simulink model "TorqueVect_FS_with_kalmanFilter"  (R2022a)
settings: Solver=FixedStepAuto  StartTime=0.0  StopTime=inf  FixedStep=0.001  RelTol=1e-3  EnableMultiTasking=on
PreLoadFcn:
  | run('Parameters\FSE_Parameters.m')
libraries: CarMaker4SL x42, simulink x1
(part 3 of 3)

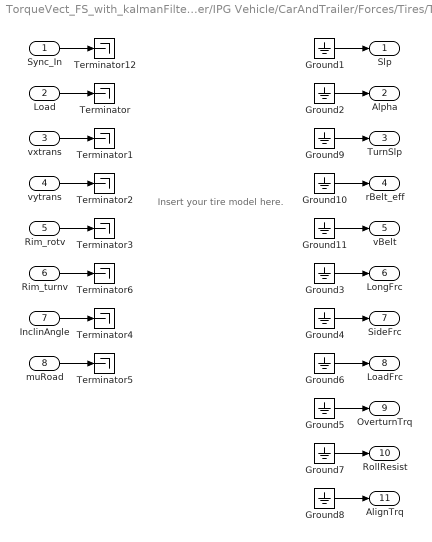
== system TorqueVect_FS_with_kalmanFilter/CarMaker/IPG Vehicle/CarAndTrailer/Forces/Tires/TireRL ==
  note: Insert your tire model here.
  Sync_In : Inport
  Load : Inport  Port=2
  vxtrans : Inport  Port=3
  vytrans : Inport  Port=4
  Rim_rotv : Inport  Port=5
  Rim_turnv : Inport  Port=6
  InclinAngle : Inport  Port=7
  muRoad : Inport  Port=8
  Ground{1..11} (11 alike) : Ground
  Terminator{,1..6,12} (8 alike) : Terminator
  Slp : Outport
  Alpha : Outport  Port=2
  TurnSlp : Outport  Port=3
  rBelt_eff : Outport  Port=4
  vBelt : Outport  Port=5
  LongFrc : Outport  Port=6
  SideFrc : Outport  Port=7
  LoadFrc : Outport  Port=8
  OverturnTrq : Outport  Port=9
  RollResist : Outport  Port=10
  AlignTrq : Outport  Port=11
  wires:
  Ground11/1 -> vBelt/1
  Ground10/1 -> rBelt_eff/1
  Ground9/1 -> TurnSlp/1
  Rim_turnv/1 -> Terminator6/1
  Sync_In/1 -> Terminator12/1
  Ground2/1 -> Alpha/1
  Ground3/1 -> LongFrc/1
  Ground4/1 -> SideFrc/1
  Ground5/1 -> OverturnTrq/1
  vxtrans/1 -> Terminator1/1
  vytrans/1 -> Terminator2/1
  Rim_rotv/1 -> Terminator3/1
  InclinAngle/1 -> Terminator4/1
  muRoad/1 -> Terminator5/1
  Load/1 -> Terminator/1
  Ground1/1 -> Slp/1
  Ground6/1 -> LoadFrc/1
  Ground7/1 -> RollResist/1
  Ground8/1 -> AlignTrq/1

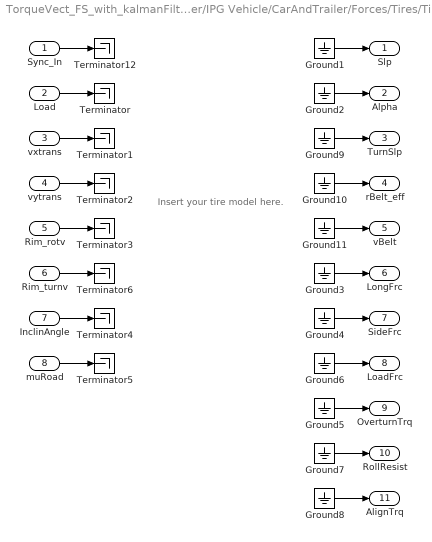
== system TorqueVect_FS_with_kalmanFilter/CarMaker/IPG Vehicle/CarAndTrailer/Forces/Tires/TireRR ==
  note: Insert your tire model here.
  Sync_In : Inport
  Load : Inport  Port=2
  vxtrans : Inport  Port=3
  vytrans : Inport  Port=4
  Rim_rotv : Inport  Port=5
  Rim_turnv : Inport  Port=6
  InclinAngle : Inport  Port=7
  muRoad : Inport  Port=8
  Ground{1..11} (11 alike) : Ground
  Terminator{,1..6,12} (8 alike) : Terminator
  Slp : Outport
  Alpha : Outport  Port=2
  TurnSlp : Outport  Port=3
  rBelt_eff : Outport  Port=4
  vBelt : Outport  Port=5
  LongFrc : Outport  Port=6
  SideFrc : Outport  Port=7
  LoadFrc : Outport  Port=8
  OverturnTrq : Outport  Port=9
  RollResist : Outport  Port=10
  AlignTrq : Outport  Port=11
  wires:
  Ground11/1 -> vBelt/1
  Ground10/1 -> rBelt_eff/1
  Ground9/1 -> TurnSlp/1
  Rim_turnv/1 -> Terminator6/1
  Sync_In/1 -> Terminator12/1
  Ground2/1 -> Alpha/1
  Ground3/1 -> LongFrc/1
  Ground4/1 -> SideFrc/1
  Ground5/1 -> OverturnTrq/1
  vxtrans/1 -> Terminator1/1
  vytrans/1 -> Terminator2/1
  Rim_rotv/1 -> Terminator3/1
  InclinAngle/1 -> Terminator4/1
  muRoad/1 -> Terminator5/1
  Load/1 -> Terminator/1
  Ground1/1 -> Slp/1
  Ground6/1 -> LoadFrc/1
  Ground7/1 -> RollResist/1
  Ground8/1 -> AlignTrq/1

== system TorqueVect_FS_with_kalmanFilter/CarMaker/IPG Vehicle/PowerTrain/PTControl Example/PTControl/Control_value ==
  ht : Inport
  lf : Inport  Port=2
  FL_Fx : Inport  Port=3
  FR_Fx : Inport  Port=4
  cos : Inport  Port=5
  sin : Inport  Port=6
  FR : Inport  Port=7
  In8 : Inport  Port=8
  Add{4..7} (4 alike) : Sum
  Minus : Sum  Inputs=+-
  Product{10..13,15..17} (7 alike) : Product
  Mx : Outport
  wires:
  Product10/1 -> Minus/1
  cos/1 -> Product10/2, Product11/1
  FR_Fx/1 -> Product13/2, Product11/2
  Product16/1 -> Add5/2
  sin/1 -> Product12/1, Product13/1
  Product17/1 -> Add5/1
  ht/1 -> Product15/1, Product17/1
  FL_Fx/1 -> Product10/1, Product12/2
  Add5/1 -> Add7/1
  Product12/1 -> Add4/1
  In8/1 -> Add6/2
  Product11/1 -> Minus/2
  Product13/1 -> Add4/2
  Product15/1 -> Add7/2
  Add4/1 -> Product16/2
  Add6/1 -> Product15/2
  Minus/1 -> Product17/2
  FR/1 -> Add6/1
  Add7/1 -> Mx/1
  lf/1 -> Product16/1

== system TorqueVect_FS_with_kalmanFilter/CarMaker/IPG Vehicle/PowerTrain/PTControl Example/PTControl/Count1 ==
  u : Inport
  cut : Inport  Port=2
  Add1 : Sum
  Delay : Delay  DelayLength=1
  MATLAB Function : MATLAB Function  TreatAsAtomicUnit=on
  Product2 : Product
  cnt : Outport
  wires:
  Add1/1 -> cnt/1, Product2/2
  Product2/1 -> Delay/1
  MATLAB Function/1(y) -> Add1/1, Product2/1
  cut/1 -> MATLAB Function/2(cut)
  Delay/1 -> Add1/2
  u/1 -> MATLAB Function/1(u)

== system TorqueVect_FS_with_kalmanFilter/CarMaker/IPG Vehicle/PowerTrain/PTControl Example/PTControl/PTC ==
  Constant2 : Constant
  Ground : Ground
  Mode_EngineDrive : Constant  Value=4
  Mux : Mux
  OperState_Driving : Constant  Value=4
  PTC MiscOut : Outport  VectorParamsAs1DForOutWhenUnconnected=off
  wires:
  Constant2/1 -> Mux/4  "Ignition"
  Mode_EngineDrive/1 -> Mux/3
  Ground/1 -> Mux/2  "OperationError"
  OperState_Driving/1 -> Mux/1
  Mux/1 -> PTC MiscOut/1

== system TorqueVect_FS_with_kalmanFilter/CarMaker/IPG Vehicle/PowerTrain/PTControl Example/PTControl_In/CreateBus PTC Battery ==
  In : Inport
  BusCreator : BusCreator  Inputs=14
  Demux : Demux  Outputs=14
      settings: DisplayOption=none
  Out : Outport  VectorParamsAs1DForOutWhenUnconnected=off
  wires:
  In/1 -> Demux/1
  BusCreator/1 -> Out/1
  Demux/1 -> BusCreator/1  "PTC BattLVIn SOC"
  Demux/2 -> BusCreator/2  "PTC BattLVIn SOH"
  Demux/3 -> BusCreator/3  "PTC BattLVIn Current"
  Demux/4 -> BusCreator/4  "PTC BattLVIn AOC"
  Demux/5 -> BusCreator/5  "PTC BattLVIn Temp"
  Demux/6 -> BusCreator/6  "PTC BattLVIn Energy"
  Demux/7 -> BusCreator/7  "PTC BattLVIn Pwr_max"
  Demux/8 -> BusCreator/8  "PTC BattHVIn SOC"
  Demux/9 -> BusCreator/9  "PTC BattHVIn SOH"
  Demux/10 -> BusCreator/10  "PTC BattHVIn Current"
  Demux/11 -> BusCreator/11  "PTC BattHVIn AOC"
  Demux/12 -> BusCreator/12  "PTC BattHVIn Temp"
  Demux/13 -> BusCreator/13  "PTC BattHVIn Energy"
  Demux/14 -> BusCreator/14  "PTC BattHVIn Pwr_max"

== system TorqueVect_FS_with_kalmanFilter/CarMaker/IPG Vehicle/PowerTrain/PTControl Example/PTControl_In/CreateBus PTC ClutchIn ==
  In : Inport
  BusCreator : BusCreator  Inputs=6
  Demux : Demux  Outputs=6
      settings: DisplayOption=none
  Out : Outport  VectorParamsAs1DForOutWhenUnconnected=off
  wires:
  In/1 -> Demux/1
  BusCreator/1 -> Out/1
  Demux/1 -> BusCreator/1  "PTC ClutchIn Pos"
  Demux/2 -> BusCreator/2  "PTC ClutchIn rotv_in"
  Demux/3 -> BusCreator/3  "PTC ClutchIn rotv_out"
  Demux/4 -> BusCreator/4  "PTC ClutchIn Trq_in"
  Demux/5 -> BusCreator/5  "PTC ClutchIn Trq_out"
  Demux/6 -> BusCreator/6  "PTC ClutchIn i_TrqIn2Out"

== system TorqueVect_FS_with_kalmanFilter/CarMaker/IPG Vehicle/PowerTrain/PTControl Example/PTControl_In/CreateBus PTC Control Units ==
  In : Inport
  BusCreator : BusCreator  Inputs=4
  Demux : Demux
      settings: DisplayOption=none
  Out : Outport  VectorParamsAs1DForOutWhenUnconnected=off
  wires:
  In/1 -> Demux/1
  BusCreator/1 -> Out/1
  Demux/1 -> BusCreator/1  "PTC ECU_Status"
  Demux/2 -> BusCreator/2  "PTC MCU_Status"
  Demux/3 -> BusCreator/3  "PTC TCU_Status"
  Demux/4 -> BusCreator/4  "PTC BCU_Status"

== system TorqueVect_FS_with_kalmanFilter/CarMaker/IPG Vehicle/PowerTrain/PTControl Example/PTControl_In/CreateBus PTC DriveSrcIn ==
  In : Inport
  BusCreator : BusCreator  Inputs=4
  Demux : Demux
      settings: DisplayOption=none
  Out : Outport  VectorParamsAs1DForOutWhenUnconnected=off
  wires:
  In/1 -> Demux/1
  BusCreator/1 -> Out/1
  Demux/1 -> BusCreator/1  "PTC DriveSrcIn_d0 Trq_DriveSrc_trg"
  Demux/2 -> BusCreator/2  "PTC DriveSrcIn_d1 Trq_DriveSrc_trg"
  Demux/3 -> BusCreator/3  "PTC DriveSrcIn_d2 Trq_DriveSrc_trg"
  Demux/4 -> BusCreator/4  "PTC DriveSrcIn_d3 Trq_DriveSrc_trg"

== system TorqueVect_FS_with_kalmanFilter/CarMaker/IPG Vehicle/PowerTrain/PTControl Example/PTControl_In/CreateBus PTC EngineIn ==
  In : Inport
  BusCreator : BusCreator  Inputs=7
  Demux : Demux  Outputs=7
      settings: DisplayOption=none
  Out : Outport  VectorParamsAs1DForOutWhenUnconnected=off
  wires:
  In/1 -> Demux/1
  BusCreator/1 -> Out/1
  Demux/1 -> BusCreator/1  "PTC EngineIn Engine_on"
  Demux/2 -> BusCreator/2  "PTC EngineIn rotv"
  Demux/3 -> BusCreator/3  "PTC EngineIn Trq"
  Demux/4 -> BusCreator/4  "PTC EngineIn TrqDrag"
  Demux/5 -> BusCreator/5  "PTC EngineIn TrqFull"
  Demux/6 -> BusCreator/6  "PTC EngineIn TrqOpt"
  Demux/7 -> BusCreator/7  "PTC EngineIn FuelFlow"

== system TorqueVect_FS_with_kalmanFilter/CarMaker/IPG Vehicle/PowerTrain/PTControl Example/PTControl_In/CreateBus PTC GearBoxIn ==
  In : Inport
  BusCreator : BusCreator  Inputs=20
  Demux : Demux  Outputs=20
      settings: DisplayOption=none
  Out : Outport  VectorParamsAs1DForOutWhenUnconnected=off
  wires:
  In/1 -> Demux/1
  BusCreator/1 -> Out/1
  Demux/1 -> BusCreator/1  "PTC GearBoxIn GearNo"
  Demux/2 -> BusCreator/2  "PTC GearBoxIn GearNo_dis"
  Demux/3 -> BusCreator/3  "PTC GearBoxIn Trq_DriveSrc_trg"
  Demux/4 -> BusCreator/4  "PTC GearBoxIn i"
  Demux/5 -> BusCreator/5  "PTC GearBoxIn rotv_in"
  Demux/6 -> BusCreator/6  "PTC GearBoxIn rotv_out"
  Demux/7 -> BusCreator/7  "PTC GearBoxIn Trq_in"
  Demux/8 -> BusCreator/8  "PTC GearBoxIn Trq_out"
  Demux/9 -> BusCreator/9  "PTC GearBoxIn Clutch Pos"
  Demux/10 -> BusCreator/10  "PTC GearBoxIn Clutch rotv_in"
  Demux/11 -> BusCreator/11  "PTC GearBoxIn Clutch rotv_out"
  Demux/12 -> BusCreator/12  "PTC GearBoxIn Clutch Trq_in"
  Demux/13 -> BusCreator/13  "PTC GearBoxIn Clutch Trq_out"
  Demux/14 -> BusCreator/14  "PTC GearBoxIn Clutch i_TrqIn2Out"
  Demux/15 -> BusCreator/15  "PTC GearBoxIn Clutch_dis Pos"
  Demux/16 -> BusCreator/16  "PTC GearBoxIn Clutch_dis rotv_in"
  Demux/17 -> BusCreator/17  "PTC GearBoxIn Clutch_dis rotv_out"
  Demux/18 -> BusCreator/18  "PTC GearBoxIn Clutch_dis Trq_in"
  Demux/19 -> BusCreator/19  "PTC GearBoxIn Clutch_dis Trq_out"
  Demux/20 -> BusCreator/20  "PTC GearBoxIn Clutch_dis i_TrqIn2Out"

== system TorqueVect_FS_with_kalmanFilter/CarMaker/IPG Vehicle/PowerTrain/PTControl Example/PTControl_In/CreateBus PTC GearBoxM_In0 ==
  In : Inport
  BusCreator : BusCreator  Inputs=20
  Demux : Demux  Outputs=20
      settings: DisplayOption=none
  Out : Outport  VectorParamsAs1DForOutWhenUnconnected=off
  wires:
  In/1 -> Demux/1
  BusCreator/1 -> Out/1
  Demux/1 -> BusCreator/1  "PTC GearBoxM_In0 GearNo"
  Demux/2 -> BusCreator/2  "PTC GearBoxM_In0 GearNo_dis"
  Demux/3 -> BusCreator/3  "PTC GearBoxM_In0 Trq_DriveSrc_trg"
  Demux/4 -> BusCreator/4  "PTC GearBoxM_In0 i"
  Demux/5 -> BusCreator/5  "PTC GearBoxM_In0 rotv_in"
  Demux/6 -> BusCreator/6  "PTC GearBoxM_In0 rotv_out"
  Demux/7 -> BusCreator/7  "PTC GearBoxM_In0 Trq_in"
  Demux/8 -> BusCreator/8  "PTC GearBoxM_In0 Trq_out"
  Demux/9 -> BusCreator/9  "PTC GearBoxM_In0 Clutch Pos"
  Demux/10 -> BusCreator/10  "PTC GearBoxM_In0 Clutch rotv_in"
  Demux/11 -> BusCreator/11  "PTC GearBoxM_In0 Clutch rotv_out"
  Demux/12 -> BusCreator/12  "PTC GearBoxM_In0 Clutch Trq_in"
  Demux/13 -> BusCreator/13  "PTC GearBoxM_In0 Clutch Trq_out"
  Demux/14 -> BusCreator/14  "PTC GearBoxM_In0 Clutch i_TrqIn2Out"
  Demux/15 -> BusCreator/15  "PTC GearBoxM_In0 Clutch_dis Pos"
  Demux/16 -> BusCreator/16  "PTC GearBoxM_In0 Clutch_dis rotv_in"
  Demux/17 -> BusCreator/17  "PTC GearBoxM_In0 Clutch_dis rotv_out"
  Demux/18 -> BusCreator/18  "PTC GearBoxM_In0 Clutch_dis Trq_in"
  Demux/19 -> BusCreator/19  "PTC GearBoxM_In0 Clutch_dis Trq_out"
  Demux/20 -> BusCreator/20  "PTC GearBoxM_In0 Clutch_dis i_TrqIn2Out"

== system TorqueVect_FS_with_kalmanFilter/CarMaker/IPG Vehicle/PowerTrain/PTControl Example/PTControl_In/CreateBus PTC GearBoxM_In1 ==
  In : Inport
  BusCreator : BusCreator  Inputs=20
  Demux : Demux  Outputs=20
      settings: DisplayOption=none
  Out : Outport  VectorParamsAs1DForOutWhenUnconnected=off
  wires:
  In/1 -> Demux/1
  BusCreator/1 -> Out/1
  Demux/1 -> BusCreator/1  "PTC GearBoxM_In1 GearNo"
  Demux/2 -> BusCreator/2  "PTC GearBoxM_In1 GearNo_dis"
  Demux/3 -> BusCreator/3  "PTC GearBoxM_In1 Trq_DriveSrc_trg"
  Demux/4 -> BusCreator/4  "PTC GearBoxM_In1 i"
  Demux/5 -> BusCreator/5  "PTC GearBoxM_In1 rotv_in"
  Demux/6 -> BusCreator/6  "PTC GearBoxM_In1 rotv_out"
  Demux/7 -> BusCreator/7  "PTC GearBoxM_In1 Trq_in"
  Demux/8 -> BusCreator/8  "PTC GearBoxM_In1 Trq_out"
  Demux/9 -> BusCreator/9  "PTC GearBoxM_In1 Clutch Pos"
  Demux/10 -> BusCreator/10  "PTC GearBoxM_In1 Clutch rotv_in"
  Demux/11 -> BusCreator/11  "PTC GearBoxM_In1 Clutch rotv_out"
  Demux/12 -> BusCreator/12  "PTC GearBoxM_In1 Clutch Trq_in"
  Demux/13 -> BusCreator/13  "PTC GearBoxM_In1 Clutch Trq_out"
  Demux/14 -> BusCreator/14  "PTC GearBoxM_In1 Clutch i_TrqIn2Out"
  Demux/15 -> BusCreator/15  "PTC GearBoxM_In1 Clutch_dis Pos"
  Demux/16 -> BusCreator/16  "PTC GearBoxM_In1 Clutch_dis rotv_in"
  Demux/17 -> BusCreator/17  "PTC GearBoxM_In1 Clutch_dis rotv_out"
  Demux/18 -> BusCreator/18  "PTC GearBoxM_In1 Clutch_dis Trq_in"
  Demux/19 -> BusCreator/19  "PTC GearBoxM_In1 Clutch_dis Trq_out"
  Demux/20 -> BusCreator/20  "PTC GearBoxM_In1 Clutch_dis i_TrqIn2Out"

== system TorqueVect_FS_with_kalmanFilter/CarMaker/IPG Vehicle/PowerTrain/PTControl Example/PTControl_In/CreateBus PTC GearBoxM_In2 ==
  In : Inport
  BusCreator : BusCreator  Inputs=20
  Demux : Demux  Outputs=20
      settings: DisplayOption=none
  Out : Outport  VectorParamsAs1DForOutWhenUnconnected=off
  wires:
  In/1 -> Demux/1
  BusCreator/1 -> Out/1
  Demux/1 -> BusCreator/1  "PTC GearBoxM_In2 GearNo"
  Demux/2 -> BusCreator/2  "PTC GearBoxM_In2 GearNo_dis"
  Demux/3 -> BusCreator/3  "PTC GearBoxM_In2 Trq_DriveSrc_trg"
  Demux/4 -> BusCreator/4  "PTC GearBoxM_In2 i"
  Demux/5 -> BusCreator/5  "PTC GearBoxM_In2 rotv_in"
  Demux/6 -> BusCreator/6  "PTC GearBoxM_In2 rotv_out"
  Demux/7 -> BusCreator/7  "PTC GearBoxM_In2 Trq_in"
  Demux/8 -> BusCreator/8  "PTC GearBoxM_In2 Trq_out"
  Demux/9 -> BusCreator/9  "PTC GearBoxM_In2 Clutch Pos"
  Demux/10 -> BusCreator/10  "PTC GearBoxM_In2 Clutch rotv_in"
  Demux/11 -> BusCreator/11  "PTC GearBoxM_In2 Clutch rotv_out"
  Demux/12 -> BusCreator/12  "PTC GearBoxM_In2 Clutch Trq_in"
  Demux/13 -> BusCreator/13  "PTC GearBoxM_In2 Clutch Trq_out"
  Demux/14 -> BusCreator/14  "PTC GearBoxM_In2 Clutch i_TrqIn2Out"
  Demux/15 -> BusCreator/15  "PTC GearBoxM_In2 Clutch_dis Pos"
  Demux/16 -> BusCreator/16  "PTC GearBoxM_In2 Clutch_dis rotv_in"
  Demux/17 -> BusCreator/17  "PTC GearBoxM_In2 Clutch_dis rotv_out"
  Demux/18 -> BusCreator/18  "PTC GearBoxM_In2 Clutch_dis Trq_in"
  Demux/19 -> BusCreator/19  "PTC GearBoxM_In2 Clutch_dis Trq_out"
  Demux/20 -> BusCreator/20  "PTC GearBoxM_In2 Clutch_dis i_TrqIn2Out"

== system TorqueVect_FS_with_kalmanFilter/CarMaker/IPG Vehicle/PowerTrain/PTControl Example/PTControl_In/CreateBus PTC GearBoxM_In3 ==
  In : Inport
  BusCreator : BusCreator  Inputs=20
  Demux : Demux  Outputs=20
      settings: DisplayOption=none
  Out : Outport  VectorParamsAs1DForOutWhenUnconnected=off
  wires:
  In/1 -> Demux/1
  BusCreator/1 -> Out/1
  Demux/1 -> BusCreator/1  "PTC GearBoxM_In3 GearNo"
  Demux/2 -> BusCreator/2  "PTC GearBoxM_In3 GearNo_dis"
  Demux/3 -> BusCreator/3  "PTC GearBoxM_In3 Trq_DriveSrc_trg"
  Demux/4 -> BusCreator/4  "PTC GearBoxM_In3 i"
  Demux/5 -> BusCreator/5  "PTC GearBoxM_In3 rotv_in"
  Demux/6 -> BusCreator/6  "PTC GearBoxM_In3 rotv_out"
  Demux/7 -> BusCreator/7  "PTC GearBoxM_In3 Trq_in"
  Demux/8 -> BusCreator/8  "PTC GearBoxM_In3 Trq_out"
  Demux/9 -> BusCreator/9  "PTC GearBoxM_In3 Clutch Pos"
  Demux/10 -> BusCreator/10  "PTC GearBoxM_In3 Clutch rotv_in"
  Demux/11 -> BusCreator/11  "PTC GearBoxM_In3 Clutch rotv_out"
  Demux/12 -> BusCreator/12  "PTC GearBoxM_In3 Clutch Trq_in"
  Demux/13 -> BusCreator/13  "PTC GearBoxM_In3 Clutch Trq_out"
  Demux/14 -> BusCreator/14  "PTC GearBoxM_In3 Clutch i_TrqIn2Out"
  Demux/15 -> BusCreator/15  "PTC GearBoxM_In3 Clutch_dis Pos"
  Demux/16 -> BusCreator/16  "PTC GearBoxM_In3 Clutch_dis rotv_in"
  Demux/17 -> BusCreator/17  "PTC GearBoxM_In3 Clutch_dis rotv_out"
  Demux/18 -> BusCreator/18  "PTC GearBoxM_In3 Clutch_dis Trq_in"
  Demux/19 -> BusCreator/19  "PTC GearBoxM_In3 Clutch_dis Trq_out"
  Demux/20 -> BusCreator/20  "PTC GearBoxM_In3 Clutch_dis i_TrqIn2Out"

== system TorqueVect_FS_with_kalmanFilter/CarMaker/IPG Vehicle/PowerTrain/PTControl Example/PTControl_In/CreateBus PTC ISGIn ==
  In : Inport
  BusCreator : BusCreator  Inputs=9
  Demux : Demux  Outputs=9
      settings: DisplayOption=none
  Out : Outport  VectorParamsAs1DForOutWhenUnconnected=off
  wires:
  In/1 -> Demux/1
  BusCreator/1 -> Out/1
  Demux/1 -> BusCreator/1  "PTC ISGIn rotv"
  Demux/2 -> BusCreator/2  "PTC ISGIn Trq"
  Demux/3 -> BusCreator/3  "PTC ISGIn TrqMot_max"
  Demux/4 -> BusCreator/4  "PTC ISGIn TrqGen_max"
  Demux/5 -> BusCreator/5  "PTC ISGIn PwrElec"
  Demux/6 -> BusCreator/6  "PTC ISGIn i_M2W_FL"
  Demux/7 -> BusCreator/7  "PTC ISGIn i_M2W_FR"
  Demux/8 -> BusCreator/8  "PTC ISGIn i_M2W_RL"
  Demux/9 -> BusCreator/9  "PTC ISGIn i_M2W_RR"

== system TorqueVect_FS_with_kalmanFilter/CarMaker/IPG Vehicle/PowerTrain/PTControl Example/PTControl_In/CreateBus PTC MotorIn0 ==
  In : Inport
  BusCreator : BusCreator  Inputs=9
  Demux : Demux  Outputs=9
      settings: DisplayOption=none
  Out : Outport  VectorParamsAs1DForOutWhenUnconnected=off
  wires:
  In/1 -> Demux/1
  BusCreator/1 -> Out/1
  Demux/1 -> BusCreator/1  "PTC MotorIn0 rotv"
  Demux/2 -> BusCreator/2  "PTC MotorIn0 Trq"
  Demux/3 -> BusCreator/3  "PTC MotorIn0 TrqMot_max"
  Demux/4 -> BusCreator/4  "PTC MotorIn0 TrqGen_max"
  Demux/5 -> BusCreator/5  "PTC MotorIn0 PwrElec"
  Demux/6 -> BusCreator/6  "PTC MotorIn0 i_M2W_FL"
  Demux/7 -> BusCreator/7  "PTC MotorIn0 i_M2W_FR"
  Demux/8 -> BusCreator/8  "PTC MotorIn0 i_M2W_RL"
  Demux/9 -> BusCreator/9  "PTC MotorIn0 i_M2W_RR"

== system TorqueVect_FS_with_kalmanFilter/CarMaker/IPG Vehicle/PowerTrain/PTControl Example/PTControl_In/CreateBus PTC MotorIn1 ==
  In : Inport
  BusCreator : BusCreator  Inputs=9
  Demux : Demux  Outputs=9
      settings: DisplayOption=none
  Out : Outport  VectorParamsAs1DForOutWhenUnconnected=off
  wires:
  In/1 -> Demux/1
  BusCreator/1 -> Out/1
  Demux/1 -> BusCreator/1  "PTC MotorIn1 rotv"
  Demux/2 -> BusCreator/2  "PTC MotorIn1 Trq"
  Demux/3 -> BusCreator/3  "PTC MotorIn1 TrqMot_max"
  Demux/4 -> BusCreator/4  "PTC MotorIn1 TrqGen_max"
  Demux/5 -> BusCreator/5  "PTC MotorIn1 PwrElec"
  Demux/6 -> BusCreator/6  "PTC MotorIn1 i_M2W_FL"
  Demux/7 -> BusCreator/7  "PTC MotorIn1 i_M2W_FR"
  Demux/8 -> BusCreator/8  "PTC MotorIn1 i_M2W_RL"
  Demux/9 -> BusCreator/9  "PTC MotorIn1 i_M2W_RR"

== system TorqueVect_FS_with_kalmanFilter/CarMaker/IPG Vehicle/PowerTrain/PTControl Example/PTControl_In/CreateBus PTC MotorIn2 ==
  In : Inport
  BusCreator : BusCreator  Inputs=9
  Demux : Demux  Outputs=9
      settings: DisplayOption=none
  Out : Outport  VectorParamsAs1DForOutWhenUnconnected=off
  wires:
  In/1 -> Demux/1
  BusCreator/1 -> Out/1
  Demux/1 -> BusCreator/1  "PTC MotorIn2 rotv"
  Demux/2 -> BusCreator/2  "PTC MotorIn2 Trq"
  Demux/3 -> BusCreator/3  "PTC MotorIn2 TrqMot_max"
  Demux/4 -> BusCreator/4  "PTC MotorIn2 TrqGen_max"
  Demux/5 -> BusCreator/5  "PTC MotorIn2 PwrElec"
  Demux/6 -> BusCreator/6  "PTC MotorIn2 i_M2W_FL"
  Demux/7 -> BusCreator/7  "PTC MotorIn2 i_M2W_FR"
  Demux/8 -> BusCreator/8  "PTC MotorIn2 i_M2W_RL"
  Demux/9 -> BusCreator/9  "PTC MotorIn2 i_M2W_RR"

== system TorqueVect_FS_with_kalmanFilter/CarMaker/IPG Vehicle/PowerTrain/PTControl Example/PTControl_In/CreateBus PTC MotorIn3 ==
  In : Inport
  BusCreator : BusCreator  Inputs=9
  Demux : Demux  Outputs=9
      settings: DisplayOption=none
  Out : Outport  VectorParamsAs1DForOutWhenUnconnected=off
  wires:
  In/1 -> Demux/1
  BusCreator/1 -> Out/1
  Demux/1 -> BusCreator/1  "PTC MotorIn3 rotv"
  Demux/2 -> BusCreator/2  "PTC MotorIn3 Trq"
  Demux/3 -> BusCreator/3  "PTC MotorIn3 TrqMot_max"
  Demux/4 -> BusCreator/4  "PTC MotorIn3 TrqGen_max"
  Demux/5 -> BusCreator/5  "PTC MotorIn3 PwrElec"
  Demux/6 -> BusCreator/6  "PTC MotorIn3 i_M2W_FL"
  Demux/7 -> BusCreator/7  "PTC MotorIn3 i_M2W_FR"
  Demux/8 -> BusCreator/8  "PTC MotorIn3 i_M2W_RL"
  Demux/9 -> BusCreator/9  "PTC MotorIn3 i_M2W_RR"

== system TorqueVect_FS_with_kalmanFilter/CarMaker/IPG Vehicle/PowerTrain/PTControl Example/PTControl_In/CreateBus PTC PwrSupplyIn ==
  In : Inport
  BusCreator : BusCreator  Inputs=12
  Demux : Demux  Outputs=12
      settings: DisplayOption=none
  Out : Outport  VectorParamsAs1DForOutWhenUnconnected=off
  wires:
  In/1 -> Demux/1
  BusCreator/1 -> Out/1
  Demux/1 -> BusCreator/1  "PTC PwrSupplyIn Pwr_LV"
  Demux/2 -> BusCreator/2  "PTC PwrSupplyIn Pwr_HV1"
  Demux/3 -> BusCreator/3  "PTC PwrSupplyIn Pwr_HV2"
  Demux/4 -> BusCreator/4  "PTC PwrSupplyIn Voltage_LV"
  Demux/5 -> BusCreator/5  "PTC PwrSupplyIn Voltage_HV1"
  Demux/6 -> BusCreator/6  "PTC PwrSupplyIn Voltage_HV2"
  Demux/7 -> BusCreator/7  "PTC PwrSupplyIn Pwr_HV1toLV"
  Demux/8 -> BusCreator/8  "PTC PwrSupplyIn Pwr_HV1toHV2"
  Demux/9 -> BusCreator/9  "PTC PwrSupplyIn Pwr_HV1toLV_max"
  Demux/10 -> BusCreator/10  "PTC PwrSupplyIn Pwr_HV1toHV2_max"
  Demux/11 -> BusCreator/11  "PTC PwrSupplyIn Eta_HV1toLV"
  Demux/12 -> BusCreator/12  "PTC PwrSupplyIn Eta_HV1toHV2"

== system TorqueVect_FS_with_kalmanFilter/CarMaker/IPG Vehicle/PowerTrain/PTControl Example/PTControl_In/CreateBus PTC Vehicle Ctrl ==
  In : Inport
  BusCreator : BusCreator  Inputs=8
  Demux : Demux  Outputs=8
      settings: DisplayOption=none
  Out : Outport  VectorParamsAs1DForOutWhenUnconnected=off
  wires:
  In/1 -> Demux/1
  BusCreator/1 -> Out/1
  Demux/1 -> BusCreator/1  "PTC Key"
  Demux/2 -> BusCreator/2  "PTC SST"
  Demux/3 -> BusCreator/3  "PTC SelectorCtrl"
  Demux/4 -> BusCreator/4  "PTC GearNoTrg"
  Demux/5 -> BusCreator/5  "PTC Clutch"
  Demux/6 -> BusCreator/6  "PTC Gas"
  Demux/7 -> BusCreator/7  "PTC Brake"
  Demux/8 -> BusCreator/8  "PTC Velocity"

== system TorqueVect_FS_with_kalmanFilter/CarMaker/IPG Vehicle/PowerTrain/PTControl Example/PTControl_In/CreateBus PTC WheelIn ==
  In : Inport
  BusCreator : BusCreator  Inputs=4
  Demux : Demux
      settings: DisplayOption=none
  Out : Outport  VectorParamsAs1DForOutWhenUnconnected=off
  wires:
  In/1 -> Demux/1
  BusCreator/1 -> Out/1
  Demux/1 -> BusCreator/1  "PTC WheelIn_FL Trq_BrakeReg_trg"
  Demux/2 -> BusCreator/2  "PTC WheelIn_FR Trq_BrakeReg_trg"
  Demux/3 -> BusCreator/3  "PTC WheelIn_RL Trq_BrakeReg_trg"
  Demux/4 -> BusCreator/4  "PTC WheelIn_RR Trq_BrakeReg_trg"

== system TorqueVect_FS_with_kalmanFilter/CarMaker/IPG Vehicle/PowerTrain/PTControl Example/PTControl_In/CreateBus PTC_Cfg Battery ==
  In : Inport
  BusCreator : BusCreator  Inputs=8
  Demux : Demux  Outputs=8
      settings: DisplayOption=none
  Out : Outport  VectorParamsAs1DForOutWhenUnconnected=off
  wires:
  In/1 -> Demux/1
  BusCreator/1 -> Out/1
  Demux/1 -> BusCreator/1  "PTC_Cfg BattLV SOC_min"
  Demux/2 -> BusCreator/2  "PTC_Cfg BattLV SOC_max"
  Demux/3 -> BusCreator/3  "PTC_Cfg BattLV Capacity"
  Demux/4 -> BusCreator/4  "PTC_Cfg BattLV Voltage"
  Demux/5 -> BusCreator/5  "PTC_Cfg BattHV SOC_min"
  Demux/6 -> BusCreator/6  "PTC_Cfg BattHV SOC_max"
  Demux/7 -> BusCreator/7  "PTC_Cfg BattHV Capacity"
  Demux/8 -> BusCreator/8  "PTC_Cfg BattHV Voltage"

== system TorqueVect_FS_with_kalmanFilter/CarMaker/IPG Vehicle/PowerTrain/PTControl Example/PTControl_In/CreateBus PTC_Cfg Engine ==
  In : Inport
  BusCreator : BusCreator  Inputs=4
  Demux : Demux
      settings: DisplayOption=none
  Out : Outport  VectorParamsAs1DForOutWhenUnconnected=off
  wires:
  In/1 -> Demux/1
  BusCreator/1 -> Out/1
  Demux/1 -> BusCreator/1  "PTC_Cfg Engine Fuel_l2kWh"
  Demux/2 -> BusCreator/2  "PTC_Cfg Engine rotv_max"
  Demux/3 -> BusCreator/3  "PTC_Cfg Engine rotv_idle"
  Demux/4 -> BusCreator/4  "PTC_Cfg Engine rotv_opt"

== system TorqueVect_FS_with_kalmanFilter/CarMaker/IPG Vehicle/PowerTrain/PTControl Example/PTControl_In/CreateBus PTC_Cfg GearBox ==
  In : Inport
  BusCreator : BusCreator  Inputs=38
  Demux : Demux  Outputs=38
      settings: DisplayOption=none
  Out : Outport  VectorParamsAs1DForOutWhenUnconnected=off
  wires:
  In/1 -> Demux/1
  BusCreator/1 -> Out/1
  Demux/1 -> BusCreator/1  "PTC_Cfg GearBox GBKind"
  Demux/2 -> BusCreator/2  "PTC_Cfg GearBox ClKind"
  Demux/3 -> BusCreator/3  "PTC_Cfg GearBox nFGears"
  Demux/4 -> BusCreator/4  "PTC_Cfg GearBox iFGear0"
  Demux/5 -> BusCreator/5  "PTC_Cfg GearBox iFGear1"
  Demux/6 -> BusCreator/6  "PTC_Cfg GearBox iFGear2"
  Demux/7 -> BusCreator/7  "PTC_Cfg GearBox iFGear3"
  Demux/8 -> BusCreator/8  "PTC_Cfg GearBox iFGear4"
  Demux/9 -> BusCreator/9  "PTC_Cfg GearBox iFGear5"
  Demux/10 -> BusCreator/10  "PTC_Cfg GearBox iFGear6"
  Demux/11 -> BusCreator/11  "PTC_Cfg GearBox iFGear7"
  Demux/12 -> BusCreator/12  "PTC_Cfg GearBox iFGear8"
  Demux/13 -> BusCreator/13  "PTC_Cfg GearBox iFGear9"
  Demux/14 -> BusCreator/14  "PTC_Cfg GearBox iFGear10"
  Demux/15 -> BusCreator/15  "PTC_Cfg GearBox iFGear11"
  Demux/16 -> BusCreator/16  "PTC_Cfg GearBox iFGear12"
  Demux/17 -> BusCreator/17  "PTC_Cfg GearBox iFGear13"
  Demux/18 -> BusCreator/18  "PTC_Cfg GearBox iFGear14"
  Demux/19 -> BusCreator/19  "PTC_Cfg GearBox iFGear15"
  Demux/20 -> BusCreator/20  "PTC_Cfg GearBox iFGear16"
  Demux/21 -> BusCreator/21  "PTC_Cfg GearBox nBGears"
  Demux/22 -> BusCreator/22  "PTC_Cfg GearBox iBGear0"
  Demux/23 -> BusCreator/23  "PTC_Cfg GearBox iBGear1"
  Demux/24 -> BusCreator/24  "PTC_Cfg GearBox iBGear2"
  Demux/25 -> BusCreator/25  "PTC_Cfg GearBox iBGear3"
  Demux/26 -> BusCreator/26  "PTC_Cfg GearBox iBGear4"
  Demux/27 -> BusCreator/27  "PTC_Cfg GearBox iBGear5"
  Demux/28 -> BusCreator/28  "PTC_Cfg GearBox iBGear6"
  Demux/29 -> BusCreator/29  "PTC_Cfg GearBox iBGear7"
  Demux/30 -> BusCreator/30  "PTC_Cfg GearBox iBGear8"
  Demux/31 -> BusCreator/31  "PTC_Cfg GearBox iBGear9"
  Demux/32 -> BusCreator/32  "PTC_Cfg GearBox iBGear10"
  Demux/33 -> BusCreator/33  "PTC_Cfg GearBox iBGear11"
  Demux/34 -> BusCreator/34  "PTC_Cfg GearBox iBGear12"
  Demux/35 -> BusCreator/35  "PTC_Cfg GearBox iBGear13"
  Demux/36 -> BusCreator/36  "PTC_Cfg GearBox iBGear14"
  Demux/37 -> BusCreator/37  "PTC_Cfg GearBox iBGear15"
  Demux/38 -> BusCreator/38  "PTC_Cfg GearBox iBGear16"

== system TorqueVect_FS_with_kalmanFilter/CarMaker/IPG Vehicle/PowerTrain/PTControl Example/PTControl_In/CreateBus PTC_Cfg GearBoxM0 ==
  In : Inport
  BusCreator : BusCreator  Inputs=38
  Demux : Demux  Outputs=38
      settings: DisplayOption=none
  Out : Outport  VectorParamsAs1DForOutWhenUnconnected=off
  wires:
  In/1 -> Demux/1
  BusCreator/1 -> Out/1
  Demux/1 -> BusCreator/1  "PTC_Cfg GearBoxM0 GBKind"
  Demux/2 -> BusCreator/2  "PTC_Cfg GearBoxM0 ClKind"
  Demux/3 -> BusCreator/3  "PTC_Cfg GearBoxM0 nFGears"
  Demux/4 -> BusCreator/4  "PTC_Cfg GearBoxM0 iFGear0"
  Demux/5 -> BusCreator/5  "PTC_Cfg GearBoxM0 iFGear1"
  Demux/6 -> BusCreator/6  "PTC_Cfg GearBoxM0 iFGear2"
  Demux/7 -> BusCreator/7  "PTC_Cfg GearBoxM0 iFGear3"
  Demux/8 -> BusCreator/8  "PTC_Cfg GearBoxM0 iFGear4"
  Demux/9 -> BusCreator/9  "PTC_Cfg GearBoxM0 iFGear5"
  Demux/10 -> BusCreator/10  "PTC_Cfg GearBoxM0 iFGear6"
  Demux/11 -> BusCreator/11  "PTC_Cfg GearBoxM0 iFGear7"
  Demux/12 -> BusCreator/12  "PTC_Cfg GearBoxM0 iFGear8"
  Demux/13 -> BusCreator/13  "PTC_Cfg GearBoxM0 iFGear9"
  Demux/14 -> BusCreator/14  "PTC_Cfg GearBoxM0 iFGear10"
  Demux/15 -> BusCreator/15  "PTC_Cfg GearBoxM0 iFGear11"
  Demux/16 -> BusCreator/16  "PTC_Cfg GearBoxM0 iFGear12"
  Demux/17 -> BusCreator/17  "PTC_Cfg GearBoxM0 iFGear13"
  Demux/18 -> BusCreator/18  "PTC_Cfg GearBoxM0 iFGear14"
  Demux/19 -> BusCreator/19  "PTC_Cfg GearBoxM0 iFGear15"
  Demux/20 -> BusCreator/20  "PTC_Cfg GearBoxM0 iFGear16"
  Demux/21 -> BusCreator/21  "PTC_Cfg GearBoxM0 nBGears"
  Demux/22 -> BusCreator/22  "PTC_Cfg GearBoxM0 iBGear0"
  Demux/23 -> BusCreator/23  "PTC_Cfg GearBoxM0 iBGear1"
  Demux/24 -> BusCreator/24  "PTC_Cfg GearBoxM0 iBGear2"
  Demux/25 -> BusCreator/25  "PTC_Cfg GearBoxM0 iBGear3"
  Demux/26 -> BusCreator/26  "PTC_Cfg GearBoxM0 iBGear4"
  Demux/27 -> BusCreator/27  "PTC_Cfg GearBoxM0 iBGear5"
  Demux/28 -> BusCreator/28  "PTC_Cfg GearBoxM0 iBGear6"
  Demux/29 -> BusCreator/29  "PTC_Cfg GearBoxM0 iBGear7"
  Demux/30 -> BusCreator/30  "PTC_Cfg GearBoxM0 iBGear8"
  Demux/31 -> BusCreator/31  "PTC_Cfg GearBoxM0 iBGear9"
  Demux/32 -> BusCreator/32  "PTC_Cfg GearBoxM0 iBGear10"
  Demux/33 -> BusCreator/33  "PTC_Cfg GearBoxM0 iBGear11"
  Demux/34 -> BusCreator/34  "PTC_Cfg GearBoxM0 iBGear12"
  Demux/35 -> BusCreator/35  "PTC_Cfg GearBoxM0 iBGear13"
  Demux/36 -> BusCreator/36  "PTC_Cfg GearBoxM0 iBGear14"
  Demux/37 -> BusCreator/37  "PTC_Cfg GearBoxM0 iBGear15"
  Demux/38 -> BusCreator/38  "PTC_Cfg GearBoxM0 iBGear16"

== system TorqueVect_FS_with_kalmanFilter/CarMaker/IPG Vehicle/PowerTrain/PTControl Example/PTControl_In/CreateBus PTC_Cfg GearBoxM1 ==
  In : Inport
  BusCreator : BusCreator  Inputs=38
  Demux : Demux  Outputs=38
      settings: DisplayOption=none
  Out : Outport  VectorParamsAs1DForOutWhenUnconnected=off
  wires:
  In/1 -> Demux/1
  BusCreator/1 -> Out/1
  Demux/1 -> BusCreator/1  "PTC_Cfg GearBoxM1 GBKind"
  Demux/2 -> BusCreator/2  "PTC_Cfg GearBoxM1 ClKind"
  Demux/3 -> BusCreator/3  "PTC_Cfg GearBoxM1 nFGears"
  Demux/4 -> BusCreator/4  "PTC_Cfg GearBoxM1 iFGear0"
  Demux/5 -> BusCreator/5  "PTC_Cfg GearBoxM1 iFGear1"
  Demux/6 -> BusCreator/6  "PTC_Cfg GearBoxM1 iFGear2"
  Demux/7 -> BusCreator/7  "PTC_Cfg GearBoxM1 iFGear3"
  Demux/8 -> BusCreator/8  "PTC_Cfg GearBoxM1 iFGear4"
  Demux/9 -> BusCreator/9  "PTC_Cfg GearBoxM1 iFGear5"
  Demux/10 -> BusCreator/10  "PTC_Cfg GearBoxM1 iFGear6"
  Demux/11 -> BusCreator/11  "PTC_Cfg GearBoxM1 iFGear7"
  Demux/12 -> BusCreator/12  "PTC_Cfg GearBoxM1 iFGear8"
  Demux/13 -> BusCreator/13  "PTC_Cfg GearBoxM1 iFGear9"
  Demux/14 -> BusCreator/14  "PTC_Cfg GearBoxM1 iFGear10"
  Demux/15 -> BusCreator/15  "PTC_Cfg GearBoxM1 iFGear11"
  Demux/16 -> BusCreator/16  "PTC_Cfg GearBoxM1 iFGear12"
  Demux/17 -> BusCreator/17  "PTC_Cfg GearBoxM1 iFGear13"
  Demux/18 -> BusCreator/18  "PTC_Cfg GearBoxM1 iFGear14"
  Demux/19 -> BusCreator/19  "PTC_Cfg GearBoxM1 iFGear15"
  Demux/20 -> BusCreator/20  "PTC_Cfg GearBoxM1 iFGear16"
  Demux/21 -> BusCreator/21  "PTC_Cfg GearBoxM1 nBGears"
  Demux/22 -> BusCreator/22  "PTC_Cfg GearBoxM1 iBGear0"
  Demux/23 -> BusCreator/23  "PTC_Cfg GearBoxM1 iBGear1"
  Demux/24 -> BusCreator/24  "PTC_Cfg GearBoxM1 iBGear2"
  Demux/25 -> BusCreator/25  "PTC_Cfg GearBoxM1 iBGear3"
  Demux/26 -> BusCreator/26  "PTC_Cfg GearBoxM1 iBGear4"
  Demux/27 -> BusCreator/27  "PTC_Cfg GearBoxM1 iBGear5"
  Demux/28 -> BusCreator/28  "PTC_Cfg GearBoxM1 iBGear6"
  Demux/29 -> BusCreator/29  "PTC_Cfg GearBoxM1 iBGear7"
  Demux/30 -> BusCreator/30  "PTC_Cfg GearBoxM1 iBGear8"
  Demux/31 -> BusCreator/31  "PTC_Cfg GearBoxM1 iBGear9"
  Demux/32 -> BusCreator/32  "PTC_Cfg GearBoxM1 iBGear10"
  Demux/33 -> BusCreator/33  "PTC_Cfg GearBoxM1 iBGear11"
  Demux/34 -> BusCreator/34  "PTC_Cfg GearBoxM1 iBGear12"
  Demux/35 -> BusCreator/35  "PTC_Cfg GearBoxM1 iBGear13"
  Demux/36 -> BusCreator/36  "PTC_Cfg GearBoxM1 iBGear14"
  Demux/37 -> BusCreator/37  "PTC_Cfg GearBoxM1 iBGear15"
  Demux/38 -> BusCreator/38  "PTC_Cfg GearBoxM1 iBGear16"

== system TorqueVect_FS_with_kalmanFilter/CarMaker/IPG Vehicle/PowerTrain/PTControl Example/PTControl_In/CreateBus PTC_Cfg GearBoxM2 ==
  In : Inport
  BusCreator : BusCreator  Inputs=38
  Demux : Demux  Outputs=38
      settings: DisplayOption=none
  Out : Outport  VectorParamsAs1DForOutWhenUnconnected=off
  wires:
  In/1 -> Demux/1
  BusCreator/1 -> Out/1
  Demux/1 -> BusCreator/1  "PTC_Cfg GearBoxM2 GBKind"
  Demux/2 -> BusCreator/2  "PTC_Cfg GearBoxM2 ClKind"
  Demux/3 -> BusCreator/3  "PTC_Cfg GearBoxM2 nFGears"
  Demux/4 -> BusCreator/4  "PTC_Cfg GearBoxM2 iFGear0"
  Demux/5 -> BusCreator/5  "PTC_Cfg GearBoxM2 iFGear1"
  Demux/6 -> BusCreator/6  "PTC_Cfg GearBoxM2 iFGear2"
  Demux/7 -> BusCreator/7  "PTC_Cfg GearBoxM2 iFGear3"
  Demux/8 -> BusCreator/8  "PTC_Cfg GearBoxM2 iFGear4"
  Demux/9 -> BusCreator/9  "PTC_Cfg GearBoxM2 iFGear5"
  Demux/10 -> BusCreator/10  "PTC_Cfg GearBoxM2 iFGear6"
  Demux/11 -> BusCreator/11  "PTC_Cfg GearBoxM2 iFGear7"
  Demux/12 -> BusCreator/12  "PTC_Cfg GearBoxM2 iFGear8"
  Demux/13 -> BusCreator/13  "PTC_Cfg GearBoxM2 iFGear9"
  Demux/14 -> BusCreator/14  "PTC_Cfg GearBoxM2 iFGear10"
  Demux/15 -> BusCreator/15  "PTC_Cfg GearBoxM2 iFGear11"
  Demux/16 -> BusCreator/16  "PTC_Cfg GearBoxM2 iFGear12"
  Demux/17 -> BusCreator/17  "PTC_Cfg GearBoxM2 iFGear13"
  Demux/18 -> BusCreator/18  "PTC_Cfg GearBoxM2 iFGear14"
  Demux/19 -> BusCreator/19  "PTC_Cfg GearBoxM2 iFGear15"
  Demux/20 -> BusCreator/20  "PTC_Cfg GearBoxM2 iFGear16"
  Demux/21 -> BusCreator/21  "PTC_Cfg GearBoxM2 nBGears"
  Demux/22 -> BusCreator/22  "PTC_Cfg GearBoxM2 iBGear0"
  Demux/23 -> BusCreator/23  "PTC_Cfg GearBoxM2 iBGear1"
  Demux/24 -> BusCreator/24  "PTC_Cfg GearBoxM2 iBGear2"
  Demux/25 -> BusCreator/25  "PTC_Cfg GearBoxM2 iBGear3"
  Demux/26 -> BusCreator/26  "PTC_Cfg GearBoxM2 iBGear4"
  Demux/27 -> BusCreator/27  "PTC_Cfg GearBoxM2 iBGear5"
  Demux/28 -> BusCreator/28  "PTC_Cfg GearBoxM2 iBGear6"
  Demux/29 -> BusCreator/29  "PTC_Cfg GearBoxM2 iBGear7"
  Demux/30 -> BusCreator/30  "PTC_Cfg GearBoxM2 iBGear8"
  Demux/31 -> BusCreator/31  "PTC_Cfg GearBoxM2 iBGear9"
  Demux/32 -> BusCreator/32  "PTC_Cfg GearBoxM2 iBGear10"
  Demux/33 -> BusCreator/33  "PTC_Cfg GearBoxM2 iBGear11"
  Demux/34 -> BusCreator/34  "PTC_Cfg GearBoxM2 iBGear12"
  Demux/35 -> BusCreator/35  "PTC_Cfg GearBoxM2 iBGear13"
  Demux/36 -> BusCreator/36  "PTC_Cfg GearBoxM2 iBGear14"
  Demux/37 -> BusCreator/37  "PTC_Cfg GearBoxM2 iBGear15"
  Demux/38 -> BusCreator/38  "PTC_Cfg GearBoxM2 iBGear16"

== system TorqueVect_FS_with_kalmanFilter/CarMaker/IPG Vehicle/PowerTrain/PTControl Example/PTControl_In/CreateBus PTC_Cfg GearBoxM3 ==
  In : Inport
  BusCreator : BusCreator  Inputs=38
  Demux : Demux  Outputs=38
      settings: DisplayOption=none
  Out : Outport  VectorParamsAs1DForOutWhenUnconnected=off
  wires:
  In/1 -> Demux/1
  BusCreator/1 -> Out/1
  Demux/1 -> BusCreator/1  "PTC_Cfg GearBoxM3 GBKind"
  Demux/2 -> BusCreator/2  "PTC_Cfg GearBoxM3 ClKind"
  Demux/3 -> BusCreator/3  "PTC_Cfg GearBoxM3 nFGears"
  Demux/4 -> BusCreator/4  "PTC_Cfg GearBoxM3 iFGear0"
  Demux/5 -> BusCreator/5  "PTC_Cfg GearBoxM3 iFGear1"
  Demux/6 -> BusCreator/6  "PTC_Cfg GearBoxM3 iFGear2"
  Demux/7 -> BusCreator/7  "PTC_Cfg GearBoxM3 iFGear3"
  Demux/8 -> BusCreator/8  "PTC_Cfg GearBoxM3 iFGear4"
  Demux/9 -> BusCreator/9  "PTC_Cfg GearBoxM3 iFGear5"
  Demux/10 -> BusCreator/10  "PTC_Cfg GearBoxM3 iFGear6"
  Demux/11 -> BusCreator/11  "PTC_Cfg GearBoxM3 iFGear7"
  Demux/12 -> BusCreator/12  "PTC_Cfg GearBoxM3 iFGear8"
  Demux/13 -> BusCreator/13  "PTC_Cfg GearBoxM3 iFGear9"
  Demux/14 -> BusCreator/14  "PTC_Cfg GearBoxM3 iFGear10"
  Demux/15 -> BusCreator/15  "PTC_Cfg GearBoxM3 iFGear11"
  Demux/16 -> BusCreator/16  "PTC_Cfg GearBoxM3 iFGear12"
  Demux/17 -> BusCreator/17  "PTC_Cfg GearBoxM3 iFGear13"
  Demux/18 -> BusCreator/18  "PTC_Cfg GearBoxM3 iFGear14"
  Demux/19 -> BusCreator/19  "PTC_Cfg GearBoxM3 iFGear15"
  Demux/20 -> BusCreator/20  "PTC_Cfg GearBoxM3 iFGear16"
  Demux/21 -> BusCreator/21  "PTC_Cfg GearBoxM3 nBGears"
  Demux/22 -> BusCreator/22  "PTC_Cfg GearBoxM3 iBGear0"
  Demux/23 -> BusCreator/23  "PTC_Cfg GearBoxM3 iBGear1"
  Demux/24 -> BusCreator/24  "PTC_Cfg GearBoxM3 iBGear2"
  Demux/25 -> BusCreator/25  "PTC_Cfg GearBoxM3 iBGear3"
  Demux/26 -> BusCreator/26  "PTC_Cfg GearBoxM3 iBGear4"
  Demux/27 -> BusCreator/27  "PTC_Cfg GearBoxM3 iBGear5"
  Demux/28 -> BusCreator/28  "PTC_Cfg GearBoxM3 iBGear6"
  Demux/29 -> BusCreator/29  "PTC_Cfg GearBoxM3 iBGear7"
  Demux/30 -> BusCreator/30  "PTC_Cfg GearBoxM3 iBGear8"
  Demux/31 -> BusCreator/31  "PTC_Cfg GearBoxM3 iBGear9"
  Demux/32 -> BusCreator/32  "PTC_Cfg GearBoxM3 iBGear10"
  Demux/33 -> BusCreator/33  "PTC_Cfg GearBoxM3 iBGear11"
  Demux/34 -> BusCreator/34  "PTC_Cfg GearBoxM3 iBGear12"
  Demux/35 -> BusCreator/35  "PTC_Cfg GearBoxM3 iBGear13"
  Demux/36 -> BusCreator/36  "PTC_Cfg GearBoxM3 iBGear14"
  Demux/37 -> BusCreator/37  "PTC_Cfg GearBoxM3 iBGear15"
  Demux/38 -> BusCreator/38  "PTC_Cfg GearBoxM3 iBGear16"

== system TorqueVect_FS_with_kalmanFilter/CarMaker/IPG Vehicle/PowerTrain/PTControl Example/PTControl_In/CreateBus PTC_Cfg ISG ==
  In : Inport
  BusCreator : BusCreator  Inputs=4
  Demux : Demux
      settings: DisplayOption=none
  Out : Outport  VectorParamsAs1DForOutWhenUnconnected=off
  wires:
  In/1 -> Demux/1
  BusCreator/1 -> Out/1
  Demux/1 -> BusCreator/1  "PTC_Cfg ISG Level"
  Demux/2 -> BusCreator/2  "PTC_Cfg ISG Ratio"
  Demux/3 -> BusCreator/3  "PTC_Cfg ISG rotv_Mot_max"
  Demux/4 -> BusCreator/4  "PTC_Cfg ISG rotv_Gen_max"

== system TorqueVect_FS_with_kalmanFilter/CarMaker/IPG Vehicle/PowerTrain/PTControl Example/PTControl_In/CreateBus PTC_Cfg Misc ==
  In : Inport
  BusCreator : BusCreator  Inputs=13
  Demux : Demux  Outputs=13
      settings: DisplayOption=none
  Out : Outport  VectorParamsAs1DForOutWhenUnconnected=off
  wires:
  In/1 -> Demux/1
  BusCreator/1 -> Out/1
  Demux/1 -> BusCreator/1  "PTC_Cfg PTKind"
  Demux/2 -> BusCreator/2  "PTC_Cfg ClKind"
  Demux/3 -> BusCreator/3  "PTC_Cfg nMotor"
  Demux/4 -> BusCreator/4  "PTC_Cfg nGearBoxM"
  Demux/5 -> BusCreator/5  "PTC_Cfg nPlanetGear"
  Demux/6 -> BusCreator/6  "PTC_Cfg Vehicle_nWheels"
  Demux/7 -> BusCreator/7  "PTC_Cfg WheelRadius"
  Demux/8 -> BusCreator/8  "PTC_Cfg Aero_Frcx"
  Demux/9 -> BusCreator/9  "PTC_Cfg DL_iDiff_mean"
  Demux/10 -> BusCreator/10  "PTC_Cfg DriveSourcePos0"
  Demux/11 -> BusCreator/11  "PTC_Cfg DriveSourcePos1"
  Demux/12 -> BusCreator/12  "PTC_Cfg DriveSourcePos2"
  Demux/13 -> BusCreator/13  "PTC_Cfg DriveSourcePos3"

== system TorqueVect_FS_with_kalmanFilter/CarMaker/IPG Vehicle/PowerTrain/PTControl Example/PTControl_In/CreateBus PTC_Cfg Motor ==
  In : Inport
  BusCreator : BusCreator  Inputs=16
  Demux : Demux  Outputs=16
      settings: DisplayOption=none
  Out : Outport  VectorParamsAs1DForOutWhenUnconnected=off
  wires:
  In/1 -> Demux/1
  BusCreator/1 -> Out/1
  Demux/1 -> BusCreator/1  "PTC_Cfg Motor0 Level"
  Demux/2 -> BusCreator/2  "PTC_Cfg Motor0 Ratio"
  Demux/3 -> BusCreator/3  "PTC_Cfg Motor0 rotv_Mot_max"
  Demux/4 -> BusCreator/4  "PTC_Cfg Motor0 rotv_Gen_max"
  Demux/5 -> BusCreator/5  "PTC_Cfg Motor1 Level"
  Demux/6 -> BusCreator/6  "PTC_Cfg Motor1 Ratio"
  Demux/7 -> BusCreator/7  "PTC_Cfg Motor1 rotv_Mot_max"
  Demux/8 -> BusCreator/8  "PTC_Cfg Motor1 rotv_Gen_max"
  Demux/9 -> BusCreator/9  "PTC_Cfg Motor2 Level"
  Demux/10 -> BusCreator/10  "PTC_Cfg Motor2 Ratio"
  Demux/11 -> BusCreator/11  "PTC_Cfg Motor2 rotv_Mot_max"
  Demux/12 -> BusCreator/12  "PTC_Cfg Motor2 rotv_Gen_max"
  Demux/13 -> BusCreator/13  "PTC_Cfg Motor3 Level"
  Demux/14 -> BusCreator/14  "PTC_Cfg Motor3 Ratio"
  Demux/15 -> BusCreator/15  "PTC_Cfg Motor3 rotv_Mot_max"
  Demux/16 -> BusCreator/16  "PTC_Cfg Motor3 rotv_Gen_max"

== system TorqueVect_FS_with_kalmanFilter/CarMaker/IPG Vehicle/PowerTrain/PTControl Example/PTControl_In/CreateBus PTC_Cfg PlanetGear ==
  In : Inport
  BusCreator : BusCreator  Inputs=1
  Demux : Demux  Outputs=1
      settings: DisplayOption=none
  Out : Outport  VectorParamsAs1DForOutWhenUnconnected=off
  wires:
  In/1 -> Demux/1
  BusCreator/1 -> Out/1
  Demux/1 -> BusCreator/1  "PTC_Cfg PlanetGear0 Ratio"

== matlab function TorqueVect_FS_with_kalmanFilter/CarMaker/IPG Vehicle/PowerTrain/PTControl Example/PTControl/Count1/MATLAB Function ==
  data: u input; y output; cut input
function y = fcn(u,cut)

if u < cut && u > -cut 
    y = 1; 
else
    y = 0;
end

== matlab function TorqueVect_FS_with_kalmanFilter/CarMaker/IPG Vehicle/PowerTrain/PTControl Example/PTControl/mean ==
  data: u input; y output
function y = fcn_mean(u)

y = mean(u);

== matlab function TorqueVect_FS_with_kalmanFilter/CarMaker/IPG Vehicle/PowerTrain/PTControl Example/PTControl/rad2deg ==
  data: u input; y output
function y = fcn_rad2deg(u)

y = rad2deg(u);

== matlab function TorqueVect_FS_with_kalmanFilter/CarMaker/IPG Vehicle/PowerTrain/PTControl Example/PTControl/M_phiy ==
  data: lf input; lr input; y output; ht input; delta input; F_yfl input; F_yfr input; F_yrl input; F_yrr input
function y = M_phiy(lf, lr, ht, delta, F_yfl, F_yfr, F_yrl, F_yrr)

y = lf*cos(delta)*(F_yfl+F_yfr) ...
    -lr*(F_yrl+F_yrr) + ht*sin(delta)*(F_yfl-F_yfr);

== matlab function TorqueVect_FS_with_kalmanFilter/CarMaker/IPG Vehicle/PowerTrain/PTControl Example/PTControl/TractionForeceALL1 ==
  data: tps input; y output
function y = TractionForceEst(tps)

if tps > 1.0
    tps = 1.0;
elseif tps < 0.0
    tps = 0.0;
end

maxTorque = 30; % [Nm]
gearRatio = 12.3;
tireRadius = 0.262; % [m]

y = tps*maxTorque*gearRatio/tireRadius;

== matlab function TorqueVect_FS_with_kalmanFilter/CarMaker/IPG Vehicle/PowerTrain/PTControl Example/PTControl/MATLAB Function1 ==
  data: v_x input; y output; delta input; L input
function y = r_des(v_x, delta, L)

y = v_x/L*delta;

== matlab function TorqueVect_FS_with_kalmanFilter/CarMaker/IPG Vehicle/PowerTrain/PTControl Example/PTControl/MATLAB Function2 ==
  data: force input; tps output
function tps = force2tps(force)

maxTorque = 30; % [Nm]
gearRatio = 12.3;
tireRadius = 0.262; % [m]

tps = force/(maxTorque*gearRatio/tireRadius);

== matlab function TorqueVect_FS_with_kalmanFilter/CarMaker/IPG Vehicle/PowerTrain/PTControl Example/PTControl/MATLAB Function3 ==
  data: force input; tps output
function tps = force2tps(force)

maxTorque = 30; % [Nm]
gearRatio = 12.3;
tireRadius = 0.262; % [m]

tps = force/(maxTorque*gearRatio/tireRadius);

== matlab function TorqueVect_FS_with_kalmanFilter/CarMaker/IPG Vehicle/PowerTrain/PTControl Example/PTControl/Trq_sum ==
  data: u input; y output
function y = trq_sum(u)

y = sum(u);

== matlab function TorqueVect_FS_with_kalmanFilter/CarMaker/IPG Vehicle/PowerTrain/PTControl Example/PTControl/Motor_to_traction ==
  data: motor input; y output
function y = TractionForceEst(motor)

maxTorque = 30; % [Nm]
gearRatio = 12.3;
tireRadius = 0.262; % [m]

if motor > maxTorque
    motor = maxTorque;
elseif motor < 0.0
    motor = 0.0;
end



y = motor*gearRatio/tireRadius;

== matlab function TorqueVect_FS_with_kalmanFilter/CarMaker/IPG Vehicle/PowerTrain/PTControl Example/PTControl/Motor_to_traction1 ==
  data: motor input; y output
function y = TractionForceEst(motor)

maxTorque = 30; % [Nm]
gearRatio = 12.3;
tireRadius = 0.262; % [m]

if motor > maxTorque
    motor = maxTorque;
elseif motor < 0.0
    motor = 0.0;
end




y = motor*gearRatio/tireRadius;

== matlab function TorqueVect_FS_with_kalmanFilter/CarMaker/IPG Vehicle/PowerTrain/PTControl Example/PTControl/overcheck ==
  data: tps input; y output; divide input
function y = Is_over(tps, divide)
temp = 0;
if tps >= abs(divide)
    temp =0 ;
elseif tps < divide
    over =tps - abs(divide);
    if divide < 0
        temp = -over;
    else 
        temp = over;
    end

end
y= temp;
